simulink model "ball_on_beam_sim_HW_08"  (R2018a)
settings: Solver=ode45  StartTime=0.0  StopTime=100  MaxStep=1  RelTol=1e-3
InitFcn:
  | ball_on_beam_param
undefined symbols (not defined in the file or in its folder): ball_on_beam_animation, ball_on_beam_ctrl, Par
settings Model: Creator=canla  LastModifiedBy=canla
settings OptimizationCC: LifeSpan=inf

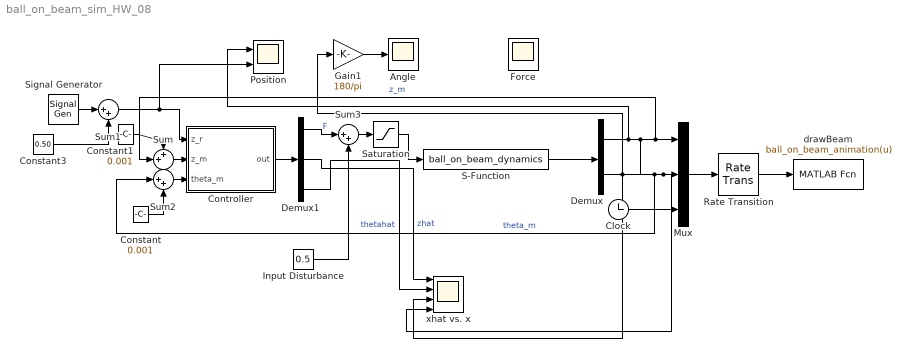
== system ball_on_beam_sim_HW_08 ==
  Angle : Scope
  Clock : Clock
  Constant : Constant  Value=0.001
  Constant1 : Constant  Value=0.001
  Constant3 : Constant  Value=0.50
  Controller : Subsystem
  Demux : Demux  Outputs=2
  Demux1 : Demux  Outputs=3
  Force : Scope
  Gain1 : Gain  Gain=180/pi
  Input Disturbance : Constant  Value=0.5
  Mux : Mux  Inputs=3
  Position : Scope  NumInputPorts=2
  Rate Transition : RateTransition  OutPortSampleTime=Par.t_plot
  S-Function : S-Function  FunctionName=ball_on_beam_dynamics  Parameters=Par  SFunctionDeploymentMode=off  EnableBusSupport=off
  Saturation : Saturate  UpperLimit=Par.F_max  LowerLimit=-Par.F_max
  Signal Generator : SignalGenerator  WaveForm=square  Amplitude=0.15  Frequency=0.025
  Sum : Sum  Inputs=++|
  Sum1 : Sum  Inputs=|++
  Sum2 : Sum  Inputs=|++
  Sum3 : Sum  Inputs=|++
  drawBeam : MATLABFcn  MATLABFcn=ball_on_beam_animation(u)  OutputDimensions=0
  xhat vs. x : Scope  NumInputPorts=4
  wires:
  Demux/2 -> Gain1/1, Sum2/1, xhat vs. x/4, Mux/2  "theta_m"
  Demux/1 -> Position/1, xhat vs. x/3, Sum/2, Mux/1  "z_m"
  Clock/1 -> Mux/3
  Mux/1 -> Rate Transition/1
  Rate Transition/1 -> drawBeam/1
  Gain1/1 -> Angle/1
  Signal Generator/1 -> Sum1/1
  Sum1/1 -> Controller/1(z_r), Position/2
  Constant3/1 -> Sum1/2
  Controller/1(out) -> Demux1/1
  Sum/1 -> Controller/2(z_m)
  Sum2/1 -> Controller/3(theta_m)
  Constant/1 -> Sum2/2
  Constant1/1 -> Sum/1
  Demux1/2 -> xhat vs. x/1  "zhat"
  Demux1/3 -> xhat vs. x/2  "thetahat"
  S-Function/1 -> Demux/1
  Saturation/1 -> S-Function/1
  Sum3/1 -> Saturation/1
  Demux1/1 -> Sum3/1  "F"
  Input Disturbance/1 -> Sum3/2

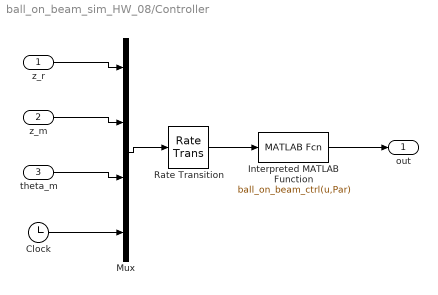
== system ball_on_beam_sim_HW_08/Controller ==
  z_r : Inport
  z_m : Inport  Port=2
  theta_m : Inport  Port=3
  Clock : Clock
  Interpreted MATLAB Function : MATLABFcn  MATLABFcn=ball_on_beam_ctrl(u,Par)
  Mux : Mux
  Rate Transition : RateTransition  OutPortSampleTime=Par.Ts
  out : Outport
  wires:
  z_r/1 -> Mux/1
  z_m/1 -> Mux/2
  theta_m/1 -> Mux/3
  Mux/1 -> Rate Transition/1
  Rate Transition/1 -> Interpreted MATLAB Function/1
  Interpreted MATLAB Function/1 -> out/1
  Clock/1 -> Mux/4
